simulink library "wind_gust_lib"  (R2015b)
settings: Solver=ode45  SolverMode=SingleTasking  StartTime=0.0  StopTime=10.0  RelTol=1e-3
undefined symbols (not defined in the file): a, b, Mq, Mw, Swg, Vto, Zw
libraries: simulink x1
settings Model: FPTRunName=Active  ModifiedByFormat=The MathWorks Inc.  ExtModeAutoUpdateStatusClock=off  Creator=The MathWorks, Inc.  LastModifiedBy=The MathWorks Inc.
settings DataIOCC: SaveFormat=Array  SignalLoggingSaveFormat=ModelDataLogs
settings OptimizationCC: BlockReduction=off  BooleanDataType=off  ExpressionDepthLimit=2147483647
settings DebuggingCC: SaveWithParameterizedLinksMsg=none  UnderspecifiedInitializationDetection=Classic  MergeDetectMultiDrivingBlocksExec=none  SignalResolutionControl=TryResolveAllWithWarning  FcnCallInpInsideContextMsg=EnableAllAsWarning  StateNameClashWarn=warning  StrictBusMsg=Warning
settings HardwareCC: ProdBitPerPointer=32  ProdLargestAtomicFloat=None  ProdIntDivRoundTo=Undefined  ProdEndianess=Unspecified  ProdWordSize=32  ProdHWDeviceType=32-bit Generic  TargetUnknown=on
settings GRTTargetCC: GeneratePreprocessorConditionals=Disable all  CombineOutputUpdateFcns=off  GRTInterface=on
settings ConfigComp: CovModelRefEnable=Off

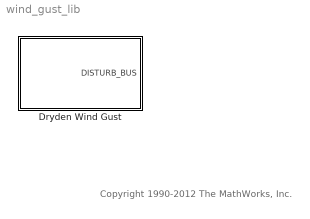
== system wind_gust_lib ==
  note: Copyright 1990-2012 The MathWorks, Inc.
  Dryden Wind Gust : Subsystem

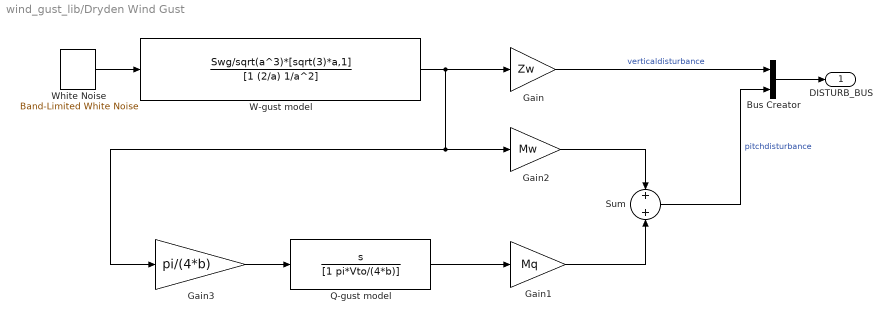
== system wind_gust_lib/Dryden Wind Gust ==
  Bus Creator : BusCreator  Inputs='verticaldisturbance','pitchdisturbance'  OutDataTypeStr=Bus: DISTURB_BUS
  Gain : Gain  Gain=Zw  SaturateOnIntegerOverflow=on  OutDataTypeStr=Inherit: Same as input  ParamDataTypeStr=Inherit: Same as input
  Gain1 : Gain  Gain=Mq  SaturateOnIntegerOverflow=on  OutDataTypeStr=Inherit: Same as input  ParamDataTypeStr=Inherit: Same as input
  Gain2 : Gain  Gain=Mw  SaturateOnIntegerOverflow=on  OutDataTypeStr=Inherit: Same as input  ParamDataTypeStr=Inherit: Same as input
  Gain3 : Gain  Gain=pi/(4*b)  SaturateOnIntegerOverflow=on  OutDataTypeStr=Inherit: Same as input  ParamDataTypeStr=Inherit: Same as input
  Q-gust model : TransferFcn  Numerator=[1 0]  Denominator=[1 pi*Vto/(4*b)]
  Sum : Sum  SaturateOnIntegerOverflow=on  InputSameDT=on  OutDataTypeStr=Inherit: Same as first input
  W-gust model : TransferFcn  Numerator=Swg/sqrt(a^3)*[sqrt(3)*a,1]  Denominator=[1 (2/a) 1/a^2]
  White Noise : simulink/Sources/Band-Limited White Noise  Cov=10  Ts=0.01  seed=23341
  DISTURB_BUS : Outport  OutDataTypeStr=Bus: DISTURB_BUS
  wires:
  Bus Creator/1 -> DISTURB_BUS/1
  Gain/1 -> Bus Creator/1  "verticaldisturbance"
  White Noise/1 -> W-gust model/1
  Gain3/1 -> Q-gust model/1
  Sum/1 -> Bus Creator/2  "pitchdisturbance"
  Gain2/1 -> Sum/1
  Gain1/1 -> Sum/2
  Q-gust model/1 -> Gain1/1
  W-gust model/1 -> Gain/1, Gain2/1, Gain3/1
